simulink model "spatiul_starilor"  (R2020a)
settings: Solver=VariableStepAuto  StartTime=0.0  StopTime=3  RelTol=1e-3
undefined symbols (not defined in the file): A, B, C, D, U
settings Model: Creator=adrian.negoita1804  LastModifiedBy=adrian.negoita1804

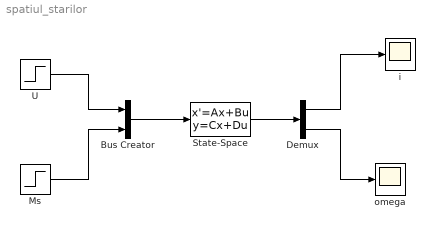
== system spatiul_starilor ==
  Bus Creator : BusCreator  Inputs=2
  Demux : Demux  Outputs=2
  Ms : Step  After=2.5  SampleTime=0
  State-Space : StateSpace  A=A  B=B  C=C  D=D  InitialCondition=0
  U : Step  After=U  SampleTime=0
  i : Scope
  omega : Scope
  wires:
  State-Space/1 -> Demux/1
  Demux/1 -> i/1
  Demux/2 -> omega/1
  Bus Creator/1 -> State-Space/1
  Ms/1 -> Bus Creator/2
  U/1 -> Bus Creator/1
